simulink library "rectifier_leg"  (R2018a)
settings: Solver=VariableStepAuto  StartTime=0.0  StopTime=10.0  RelTol=1e-3
libraries: powerlib x10
settings Model: Creator=AL-MOSTAFA  LastModifiedBy=AL-MOSTAFA

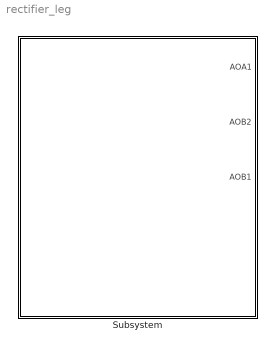
== system rectifier_leg ==
  Subsystem : Subsystem

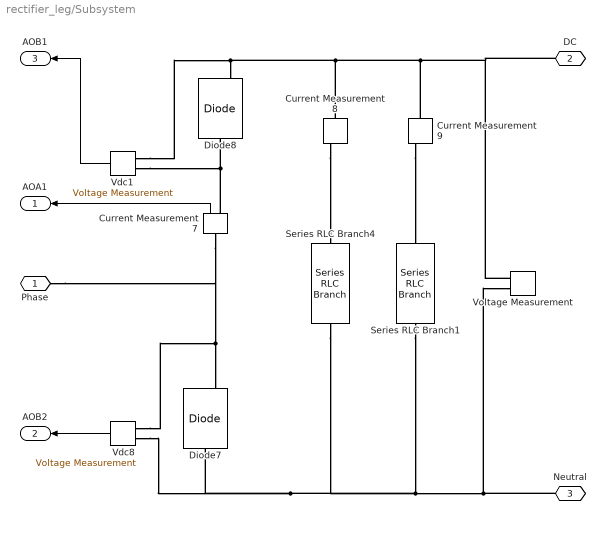
== system rectifier_leg/Subsystem ==
  Current Measurement7 : powerlib/Measurements/Current Measurement  PhasorSimulation=off  OutputType=Complex  PSBequivalent=0
  Current Measurement8 : powerlib/Measurements/Current Measurement  PhasorSimulation=off  OutputType=Complex  PSBequivalent=0
  Current Measurement9 : powerlib/Measurements/Current Measurement  PhasorSimulation=off  OutputType=Complex  PSBequivalent=0
  Diode7 : powerlib/Power Electronics/Diode  Ron=0.001  Lon=0  Vf=0.8  IC=0  UseSnubber=0  Rs=500  Cs=250e-9  Measurements=on
  Diode8 : powerlib/Power Electronics/Diode  Ron=0.001  Lon=0  Vf=0.8  IC=0  UseSnubber=0  Rs=500  Cs=250e-9  Measurements=on
  Series RLC Branch1 : powerlib/Elements/Series RLC Branch  LConnTagsString=__new0  RConnTagsString=__new0  BranchType=C  Resistance=10  Inductance=1e-3  SetiL0=off  InitialCurrent=0  Capacitance=500*10^-6  Setx0=off  InitialVoltage=0  Measurements=None
  Series RLC Branch4 : powerlib/Elements/Series RLC Branch  LConnTagsString=__new0  RConnTagsString=__new0  BranchType=C  Resistance=10  Inductance=1e-3  SetiL0=off  InitialCurrent=0  Capacitance=500*10^-6  Setx0=off  InitialVoltage=0  Measurements=None
  Vdc1 : powerlib/Measurements/Voltage Measurement  PhasorSimulation=off  OutputType=Complex  PSBequivalent=0
  Vdc8 : powerlib/Measurements/Voltage Measurement  PhasorSimulation=off  OutputType=Complex  PSBequivalent=0
  Voltage Measurement : powerlib/Measurements/Voltage Measurement  PhasorSimulation=off  OutputType=Complex  PSBequivalent=0
  Phase : PMIOPort  Side=Left
  DC : PMIOPort  Port=2  Side=Right
  Neutral : PMIOPort  Port=3  Side=Right
  AOA1 : Outport
  AOB2 : Outport  Port=2
  AOB1 : Outport  Port=3
  wires:
  Current Measurement7/1 -> AOA1/1
  Vdc8/1 -> AOB2/1
  Vdc1/1 -> AOB1/1
  connections:
  Vdc8/LConn2 -- Phase/RConn1 -- Current Measurement7/LConn1 -- Diode7/RConn1
  Current Measurement7/RConn1 -- Vdc1/LConn1 -- Diode8/LConn1
  Current Measurement8/LConn1 -- Voltage Measurement/LConn1 -- DC/RConn1 -- Current Measurement9/LConn1 -- Vdc1/LConn2 -- Diode8/RConn1
  Series RLC Branch1/RConn1 -- Series RLC Branch4/RConn1 -- Vdc8/LConn1 -- Diode7/LConn1 -- Neutral/RConn1 -- Voltage Measurement/LConn2
  Current Measurement9/RConn1 -- Series RLC Branch1/LConn1
  Current Measurement8/RConn1 -- Series RLC Branch4/LConn1
